simulink model "sampleModel1954_5_sub_sub"  (R2023a)
settings: Solver=VariableStepAuto  StartTime=0.0  StopTime=10.0  RelTol=1e-3
libraries: hdlsllib x1, simulink x1
settings Model: Creator=user1  LastModifiedBy=user1

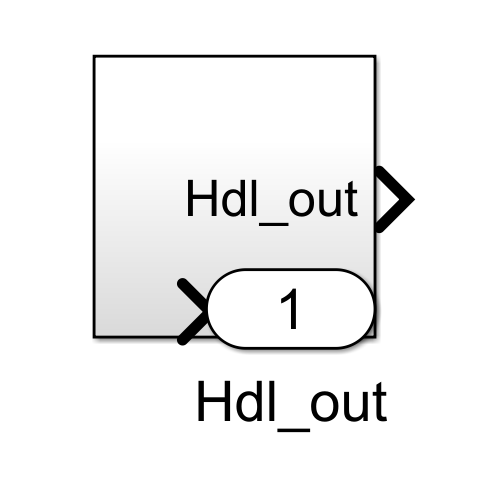
[thumbnail: Simulink's stored preview of the top-level diagram]
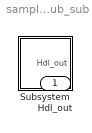
== system sampleModel1954_5_sub_sub ==
  Subsystem : Subsystem
  Hdl_out : Outport  OutDataTypeStr=uint8

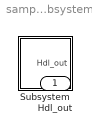
== system sampleModel1954_5_sub_sub/Subsystem ==
  Subsystem : Subsystem
  Hdl_out : Outport  OutDataTypeStr=uint8

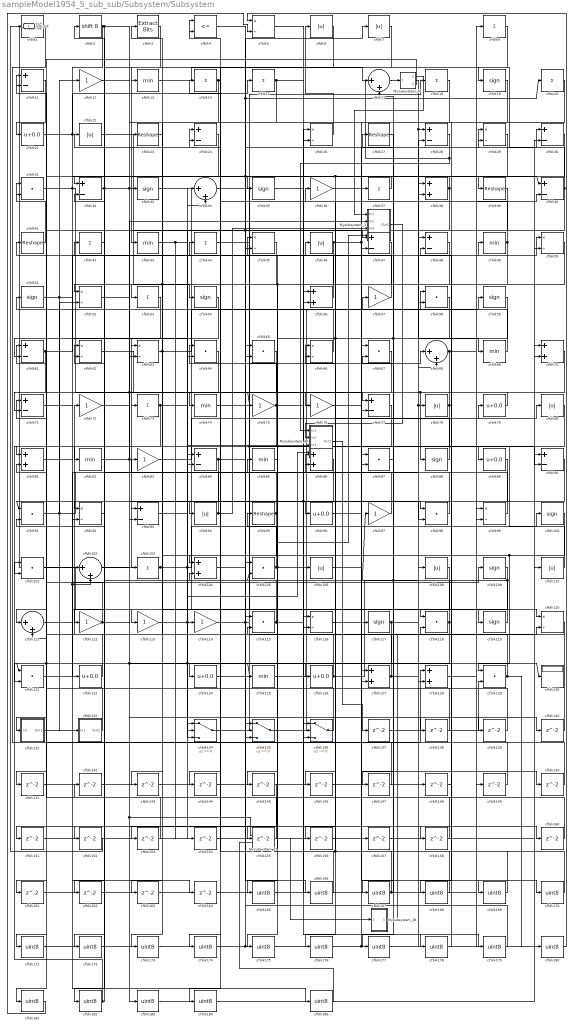
== system sampleModel1954_5_sub_sub/Subsystem/Subsystem ==
  Mysubsystem_1 : Subsystem  TreatAsAtomicUnit=on  RTWFcnName=Mysubsystem_1
      settings: RTWFcnNameOpts=User specified  RTWFileNameOpts=Use function name
  Mysubsystem_21 : Subsystem  TreatAsAtomicUnit=on  RTWFcnName=Mysubsystem_21
      settings: RTWFcnNameOpts=User specified  RTWFileNameOpts=Use function name
  Mysubsystem_38 : Subsystem  TreatAsAtomicUnit=on  RTWFcnName=Mysubsystem_38
      settings: RTWFcnNameOpts=User specified  RTWFileNameOpts=Use function name
  Mysubsystem_40 : Subsystem  TreatAsAtomicUnit=on  RTWFcnName=Mysubsystem_40
      settings: RTWFcnNameOpts=User specified  RTWFileNameOpts=Use function name
  Mysubsystem_41 : Subsystem  TreatAsAtomicUnit=on  RTWFcnName=Mysubsystem_41
      settings: RTWFcnNameOpts=User specified  RTWFileNameOpts=Use function name
  cfblk1 : hdlsllib/Logic and Bit Operations/Detect Fall Nonpositive  vinit=0  OutDataTypeStr=uint8
  cfblk{19,33,35,51,54,59,88,100,109,117,119} (11 alike) : Signum
  cfblk{31,58,64..65,67,87,91,98,101,105,115,118,121,129} (14 alike) : DotProduct  OutDataTypeStr=uint8
  cfblk{17,34,68,102,111} (5 alike) : Sum  Inputs=|++  OutDataTypeStr=uint8
  cfblk{9,14..15,18,20,37,42,44,53,73,103} (11 alike) : Sum  Inputs=+  OutDataTypeStr=uint8
  cfblk{38,56,70,81,86,104,127..128} (8 alike) : Sum  OutDataTypeStr=uint8
  cfblk{6..7,22,46,78,80,94,106,108,110} (10 alike) : Abs  OutDataTypeStr=uint8  SaturateOnIntegerOverflow=off
  cfblk{11,24,28,30,32,40,47..48,61,71,77,84,90,93} (14 alike) : Sum  Inputs=+-  OutDataTypeStr=uint8
  cfblk{12,36,57,72,75..76,83,97,112..114} (11 alike) : Gain  OutDataTypeStr=uint8
  cfblk{5,26,29,45,50,52,62..63,66,92,99,116,120} (13 alike) : Product  Inputs=*/  OutDataTypeStr=uint8  RndMeth=Zero  SaturateOnIntegerOverflow=on
  cfblk{21,79,89,96,122,124,126} (7 alike) : Bias  Bias=0.0  SaturateOnIntegerOverflow=off
  cfblk{13,43,49,69,74,82,85,125} (8 alike) : MinMax  OutDataTypeStr=uint8
  cfblk130 : Display
  cfblk131 : Subsystem
      settings: LibrarySourceBlock=|
      | hdlsllib/Ports &
      | Subsystems/Subsystem
  cfblk132 : Subsystem
      settings: LibrarySourceBlock=|
      | hdlsllib/Ports &
      | Subsystems/Subsystem
  cfblk134 : Switch  OutDataTypeStr=uint8  SaturateOnIntegerOverflow=off  InputSameDT=off
  cfblk135 : Switch  OutDataTypeStr=uint8  SaturateOnIntegerOverflow=off  InputSameDT=off
  cfblk136 : Switch  OutDataTypeStr=uint8  SaturateOnIntegerOverflow=off  InputSameDT=off
  cfblk{137..158,160..164} (27 alike) : Delay  SampleTime=1
  cfblk{165..184,186} (21 alike) : DataTypeConversion  OutDataTypeStr=uint8  SaturateOnIntegerOverflow=off  RndMeth=Floor
  cfblk2 : ArithShift  BitShiftNumber=8
  cfblk{23,27,39,41,95} (5 alike) : Reshape
  cfblk3 : simulink/Logic and Bit Operations/Extract Bits  bitsToExtract=Upper half  numBits=8  bitIdxRange=[0 7]  outScalingMode=Preserve fixed-point scaling
      settings: LibrarySourceBlock=|
      | hdlsllib/Logic and Bit
      | Operations/Extract Bits
  cfblk4 : RelationalOperator  Operator=<=  OutDataTypeStr=boolean  InputSameDT=off
  Hdl_out : Outport  OutDataTypeStr=uint8
  wires:
  Mysubsystem_41/2(Out2) -> cfblk141/1
  Mysubsystem_41/1(Out1) -> Mysubsystem_1/1(In1)
  Mysubsystem_40/1(Out1) -> cfblk137/1
  cfblk93/1 -> Mysubsystem_40/3(In3)
  Mysubsystem_1/1(Out1) -> Mysubsystem_40/2(In2)
  Mysubsystem_38/1(Out1) -> cfblk115/2
  Mysubsystem_21/1(Out1) -> Mysubsystem_38/1(In1)
  cfblk186/1 -> Mysubsystem_21/2(In2)
  cfblk184/1 -> cfblk70/2
  cfblk183/1 -> cfblk70/1
  cfblk52/1 -> cfblk183/1
  cfblk182/1 -> cfblk142/1, cfblk101/1
  cfblk181/1 -> cfblk5/2
  cfblk145/1 -> cfblk181/1
  cfblk180/1 -> cfblk5/1
  cfblk179/1 -> cfblk115/1
  cfblk5/1 -> cfblk179/1
  cfblk178/1 -> cfblk48/2
  cfblk177/1 -> cfblk48/1
  cfblk87/1 -> cfblk177/1
  cfblk176/1 -> cfblk149/1
  cfblk48/1 -> cfblk176/1
  cfblk175/1 -> cfblk9/1
  cfblk174/1 -> cfblk157/1, cfblk110/1
  cfblk173/1 -> cfblk65/2
  cfblk172/1 -> cfblk65/1
  cfblk171/1 -> cfblk148/1, cfblk135/1
  cfblk170/1 -> cfblk36/1
  cfblk96/1 -> cfblk170/1
  cfblk169/1 -> cfblk56/1
  cfblk36/1 -> cfblk169/1
  cfblk168/1 -> cfblk27/1
  cfblk19/1 -> cfblk168/1
  cfblk167/1 -> cfblk46/1, cfblk14/1, cfblk67/2
  cfblk166/1 -> cfblk85/1
  cfblk165/1 -> cfblk108/1
  cfblk85/1 -> cfblk165/1
  cfblk164/1 -> cfblk26/2
  cfblk131/1(Out1) -> cfblk164/1
  cfblk163/1 -> cfblk99/2
  cfblk162/1 -> cfblk105/1
  cfblk24/1 -> cfblk162/1
  cfblk161/1 -> cfblk128/2
  cfblk160/1 -> cfblk66/2
  cfblk12/1 -> cfblk160/1
  cfblk158/1 -> cfblk111/2
  cfblk157/1 -> cfblk30/2
  cfblk156/1 -> cfblk50/2
  cfblk155/1 -> cfblk84/1
  cfblk90/1 -> cfblk155/1
  cfblk154/1 -> cfblk127/1
  cfblk153/1 -> cfblk32/2
  cfblk20/1 -> cfblk153/1
  cfblk152/1 -> cfblk1/1
  cfblk151/1 -> cfblk134/1
  cfblk150/1 -> cfblk86/2
  cfblk149/1 -> cfblk31/2
  cfblk148/1 -> cfblk118/2
  cfblk147/1 -> cfblk62/2
  cfblk146/1 -> cfblk38/1
  cfblk58/1 -> cfblk145/1
  cfblk144/1 -> cfblk45/2
  cfblk143/1 -> cfblk56/2
  cfblk108/1 -> cfblk143/1
  cfblk142/1 -> cfblk77/2
  cfblk141/1 -> cfblk34/2
  cfblk140/1 -> cfblk11/2
  cfblk139/1 -> cfblk81/2
  cfblk138/1 -> cfblk116/1
  cfblk137/1 -> cfblk129/2
  cfblk99/1 -> cfblk62/1
  cfblk84/1 -> cfblk111/1, cfblk29/1
  cfblk66/1 -> cfblk51/1
  cfblk117/1 -> cfblk100/1, cfblk121/2
  cfblk109/1 -> cfblk105/2, cfblk124/1
  cfblk92/1 -> cfblk42/1
  cfblk91/1 -> cfblk28/2, cfblk52/2
  cfblk86/1 -> cfblk116/2
  cfblk17/1 -> cfblk28/1, cfblk69/1
  cfblk128/1 -> cfblk99/1
  cfblk56/1 -> cfblk41/1
  cfblk62/1 -> cfblk117/1
  cfblk3/1 -> cfblk13/1
  cfblk57/1 -> cfblk24/2
  cfblk125/1 -> cfblk90/1
  cfblk72/1 -> cfblk44/1
  cfblk39/1 -> cfblk135/2, cfblk151/1
  cfblk69/1 -> cfblk4/1
  cfblk46/1 -> cfblk29/2, cfblk150/1, cfblk152/1
  cfblk38/1 -> cfblk35/1, cfblk134/2
  cfblk63/1 -> cfblk58/1, cfblk173/1
  cfblk15/1 -> cfblk23/1, cfblk90/2
  cfblk64/1 -> cfblk121/1, cfblk161/1
  cfblk53/1 -> cfblk61/2
  cfblk9/1 -> cfblk174/1
  cfblk80/1 -> cfblk93/2
  cfblk105/1 -> Mysubsystem_1/4(In4), cfblk106/1, cfblk95/1
  cfblk111/1 -> cfblk86/1
  cfblk41/1 -> cfblk31/1
  cfblk71/1 -> cfblk113/1, cfblk102/2
  cfblk102/1 -> cfblk130/1, cfblk140/1
  cfblk14/1 -> cfblk63/2, cfblk144/1
  cfblk97/1 -> cfblk45/1
  cfblk100/1 -> cfblk129/1, cfblk134/3
  cfblk18/1 -> cfblk127/2
  cfblk112/1 -> cfblk11/1, cfblk138/1
  cfblk75/1 -> cfblk131/1(In1), cfblk4/2, cfblk178/1
  cfblk47/1 -> cfblk93/1
  cfblk27/1 -> cfblk167/1
  cfblk127/1 -> cfblk83/1, cfblk30/1
  cfblk116/1 -> cfblk37/1
  cfblk88/1 -> cfblk66/1
  cfblk61/1 -> cfblk71/2, cfblk50/1
  cfblk45/1 -> cfblk94/1
  cfblk136/1 -> cfblk102/1
  cfblk101/1 -> cfblk118/1
  cfblk95/1 -> cfblk24/1, cfblk163/1
  cfblk98/1 -> cfblk3/1
  cfblk79/1 -> cfblk73/1
  cfblk54/1 -> cfblk103/1
  cfblk21/1 -> cfblk38/2, cfblk15/1
  cfblk78/1 -> cfblk76/1, cfblk126/1
  cfblk113/1 -> Mysubsystem_40/4(In4), cfblk139/1
  cfblk6/1 -> cfblk32/1
  cfblk104/1 -> cfblk20/1, cfblk7/1
  cfblk65/1 -> cfblk171/1
  cfblk77/1 -> cfblk84/2
  cfblk44/1 -> cfblk87/2
  cfblk106/1 -> cfblk47/2
  cfblk30/1 -> cfblk81/1, cfblk96/1
  cfblk132/1(Out1) -> cfblk61/1
  cfblk37/1 -> cfblk33/1
  cfblk43/1 -> cfblk125/1, cfblk135/3, cfblk154/1
  cfblk23/1 -> cfblk53/1
  cfblk118/1 -> cfblk17/2, cfblk156/1
  cfblk73/1 -> cfblk49/1, cfblk101/2
  cfblk42/1 -> cfblk82/1
  cfblk115/1 -> cfblk26/1, cfblk91/2
  cfblk103/1 -> cfblk78/1, cfblk58/2, cfblk34/1, Hdl_out/1
  cfblk1/1 -> cfblk128/1
  cfblk31/1 -> cfblk114/1, cfblk186/1
  cfblk121/1 -> cfblk109/1
  cfblk59/1 -> cfblk136/2, cfblk146/1, cfblk147/1
  cfblk22/1 -> cfblk67/1
  cfblk13/1 -> cfblk17/1
  cfblk122/1 -> cfblk71/1
  cfblk81/1 -> cfblk122/1
  cfblk126/1 -> cfblk68/2, cfblk64/1
  cfblk7/1 -> cfblk43/1
  cfblk135/1 -> cfblk59/1
  cfblk4/1 -> cfblk40/1, cfblk166/1
  cfblk76/1 -> cfblk87/1
  cfblk28/1 -> Mysubsystem_41/1(In1), Mysubsystem_40/1(In1)
  cfblk110/1 -> cfblk89/1
  cfblk49/1 -> cfblk22/1, cfblk52/1
  cfblk70/1 -> cfblk182/1
  cfblk68/1 -> cfblk88/1, cfblk184/1, cfblk40/2
  cfblk129/1 -> cfblk104/2, cfblk180/1
  cfblk35/1 -> cfblk47/1
  cfblk50/1 -> cfblk63/1, cfblk92/1, cfblk175/1
  cfblk82/1 -> Mysubsystem_1/2(In2), cfblk158/1, Mysubsystem_21/1(In1)
  cfblk89/1 -> cfblk91/1, cfblk136/3
  cfblk124/1 -> cfblk120/2
  cfblk119/1 -> cfblk97/1, cfblk57/1
  cfblk2/1 -> cfblk112/1, cfblk98/2, cfblk92/2
  cfblk67/1 -> cfblk74/1
  cfblk134/1 -> cfblk18/1
  cfblk51/1 -> cfblk132/1(In1), cfblk12/1, cfblk64/2
  cfblk94/1 -> Mysubsystem_1/3(In3), cfblk2/1
  cfblk83/1 -> cfblk80/1
  cfblk32/1 -> cfblk75/1, cfblk98/1, cfblk54/1, cfblk172/1
  cfblk34/1 -> cfblk77/1
  cfblk120/1 -> cfblk72/1
  cfblk74/1 -> cfblk120/1, cfblk136/1
  cfblk29/1 -> cfblk39/1
  cfblk114/1 -> cfblk68/1, cfblk79/1
  cfblk40/1 -> cfblk19/1, cfblk104/1
  cfblk33/1 -> cfblk119/1
  cfblk11/1 -> cfblk21/1
  cfblk26/1 -> cfblk6/1

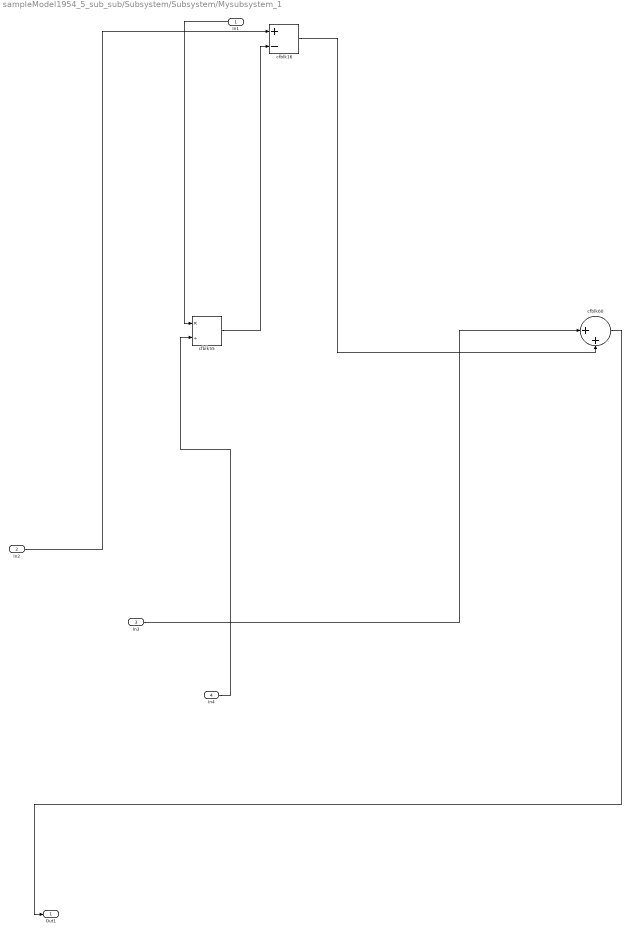
== system sampleModel1954_5_sub_sub/Subsystem/Subsystem/Mysubsystem_1 ==
  In1 : Inport
  In2 : Inport  Port=2
  In3 : Inport  Port=3
  In4 : Inport  Port=4
  cfblk16 : Sum  Inputs=+-
  cfblk55 : Product  Inputs=*/  RndMeth=Zero  SaturateOnIntegerOverflow=on
  cfblk60 : Sum  Inputs=|++
  Out1 : Outport
  wires:
  In2/1 -> cfblk16/1
  cfblk55/1 -> cfblk16/2
  cfblk16/1 -> cfblk60/2
  In3/1 -> cfblk60/1
  cfblk60/1 -> Out1/1
  In1/1 -> cfblk55/1
  In4/1 -> cfblk55/2

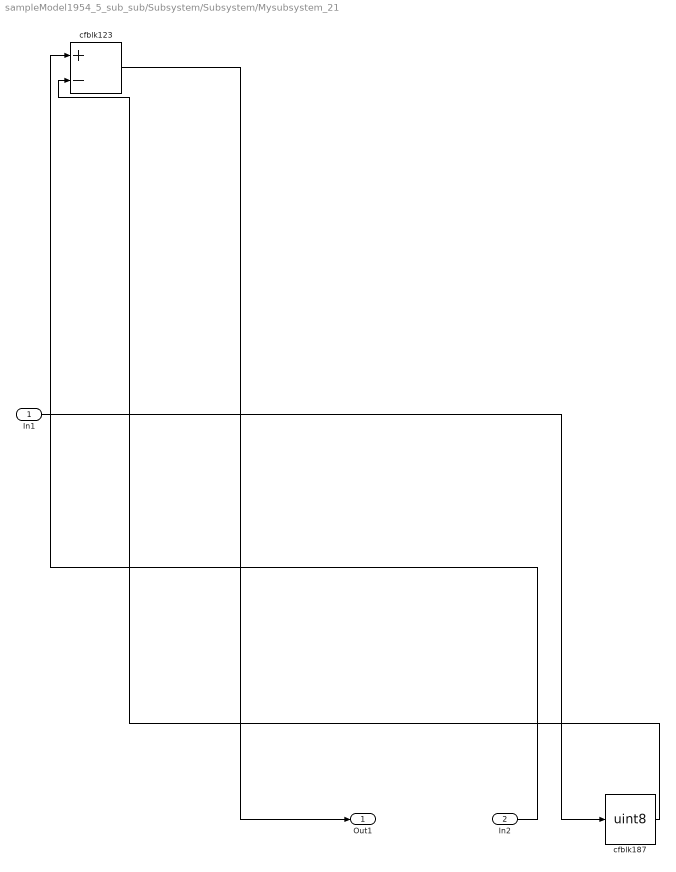
== system sampleModel1954_5_sub_sub/Subsystem/Subsystem/Mysubsystem_21 ==
  In1 : Inport
  In2 : Inport  Port=2
  cfblk123 : Sum  Inputs=+-
  cfblk187 : DataTypeConversion  OutDataTypeStr=uint8  SaturateOnIntegerOverflow=off  RndMeth=Floor
  Out1 : Outport
  wires:
  cfblk123/1 -> Out1/1
  cfblk187/1 -> cfblk123/2
  In1/1 -> cfblk187/1
  In2/1 -> cfblk123/1

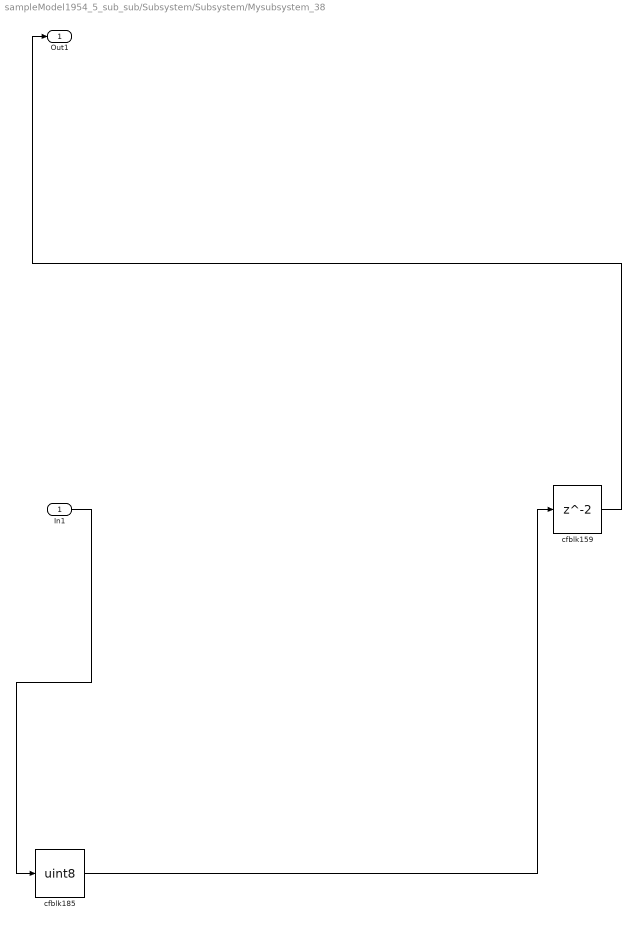
== system sampleModel1954_5_sub_sub/Subsystem/Subsystem/Mysubsystem_38 ==
  In1 : Inport
  cfblk159 : Delay  SampleTime=1
  cfblk185 : DataTypeConversion  OutDataTypeStr=uint8  SaturateOnIntegerOverflow=off  RndMeth=Floor
  Out1 : Outport
  wires:
  cfblk159/1 -> Out1/1
  cfblk185/1 -> cfblk159/1
  In1/1 -> cfblk185/1

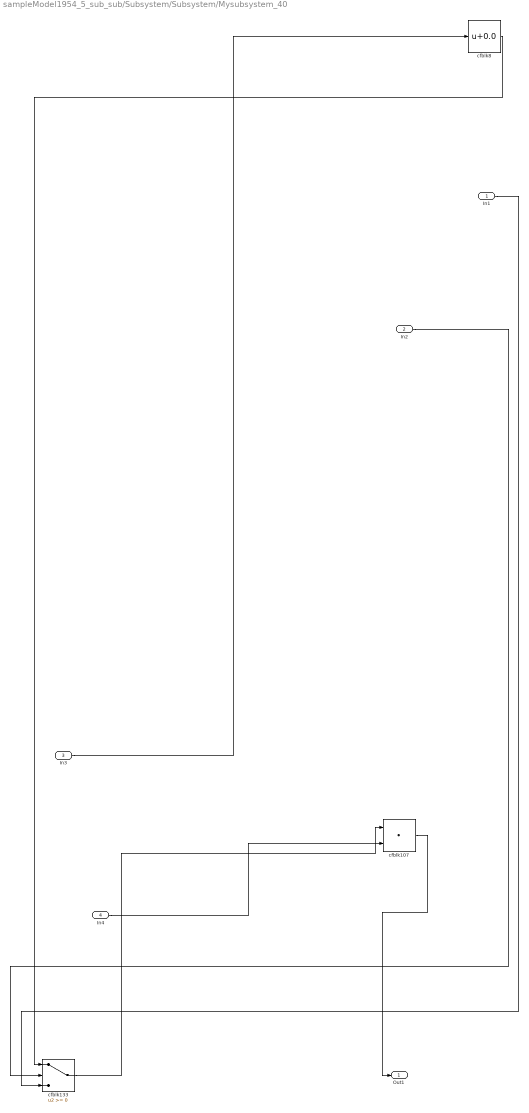
== system sampleModel1954_5_sub_sub/Subsystem/Subsystem/Mysubsystem_40 ==
  In1 : Inport
  In2 : Inport  Port=2
  In3 : Inport  Port=3
  In4 : Inport  Port=4
  cfblk107 : DotProduct  OutDataTypeStr=Inherit: Inherit via internal rule
  cfblk133 : Switch  SaturateOnIntegerOverflow=off  InputSameDT=off
  cfblk8 : Bias  Bias=0.0  SaturateOnIntegerOverflow=off
  Out1 : Outport
  wires:
  cfblk133/1 -> cfblk107/1
  cfblk8/1 -> cfblk133/1
  In2/1 -> cfblk133/2
  cfblk107/1 -> Out1/1
  In3/1 -> cfblk8/1
  In1/1 -> cfblk133/3
  In4/1 -> cfblk107/2

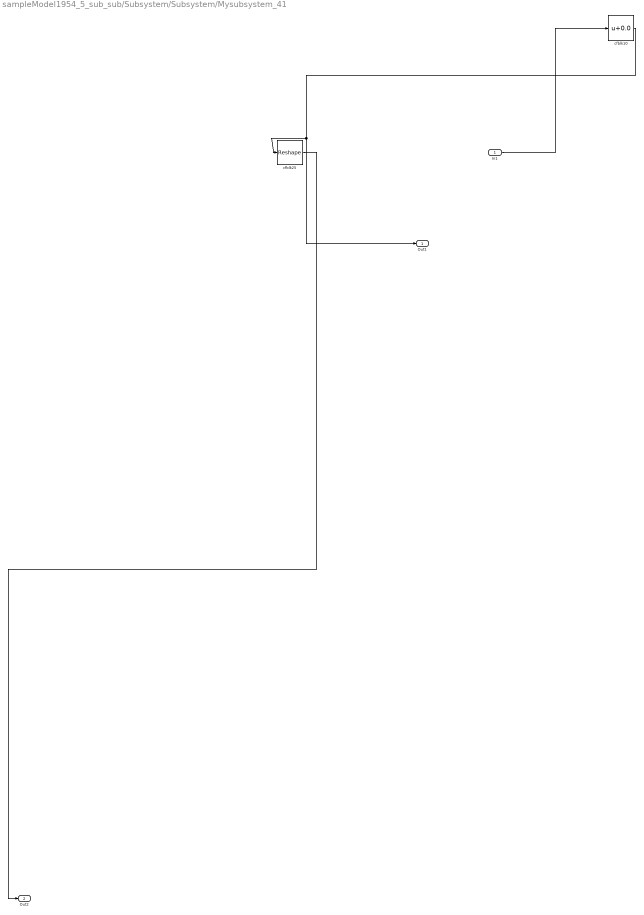
== system sampleModel1954_5_sub_sub/Subsystem/Subsystem/Mysubsystem_41 ==
  In1 : Inport
  cfblk10 : Bias  Bias=0.0  SaturateOnIntegerOverflow=off
  cfblk25 : Reshape
  Out1 : Outport
  Out2 : Outport  Port=2
  wires:
  cfblk10/1 -> Out1/1, cfblk25/1
  cfblk25/1 -> Out2/1
  In1/1 -> cfblk10/1

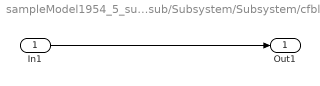
== system sampleModel1954_5_sub_sub/Subsystem/Subsystem/cfblk131 ==
  In1 : Inport
  Out1 : Outport
  wires:
  In1/1 -> Out1/1

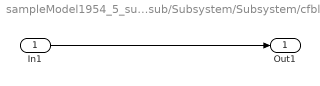
== system sampleModel1954_5_sub_sub/Subsystem/Subsystem/cfblk132 ==
  In1 : Inport
  Out1 : Outport
  wires:
  In1/1 -> Out1/1
